simulink model "simple_line_follower_simulation_new"  (R2020a)
settings: Solver=FixedStepAuto  StartTime=0.0  StopTime=5  FixedStep=0.01  RelTol=1e-3
values from neighbouring files (symbols this model uses):
  axleLength = 0.0672    [robotParameters_maze.m]
  J = 0.0001    [robotParameters_maze.m]
  Kb = 0.190    (= 0.19)    [robotParameters_maze.m]
  Kf = 0.000025    (= 2.5e-05)    [robotParameters_maze.m]
  Km = 0.084    [robotParameters_maze.m]
  L = 0.5    [robotParameters_maze.m]
  mapForSim =     [maze_map.mat]    (also in oval_line_map.mat)
  motorIP = [-12 -11.9 -11.8 -11.7 -11.6 -11.5 -11.4 -11.3 -11.2 -11.1 -11 -10.9 ... (241 elements, 1x241)]    [motorLUT.mat]
  motorSP = [-62.7865560716 -62.2538153955 -61.7309054619 -61.2077148683 -60.684548166 -60.1613790322 -59.6382101464 -59.1150412352 -58.5918723266 -58.0687034178 -57.545534509 -57.0223656001 ... (241 elements, 1x241)]    [motorLUT.mat]
  R = 16    [robotParameters_maze.m]
  wheelR = 0.017    [robotParameters_maze.m]
undefined symbols (not defined in the file or in its folder): DiscIntNeverNeededParam, lineLength
libraries: mobileRoboticsTrainingLib x2, eeGeneralControl x1, simulink x1, sldrtlib x1
settings Model: Creator=RAJENDRA PHUTANE  LastModifiedBy=RAJENDRA PHUTANE

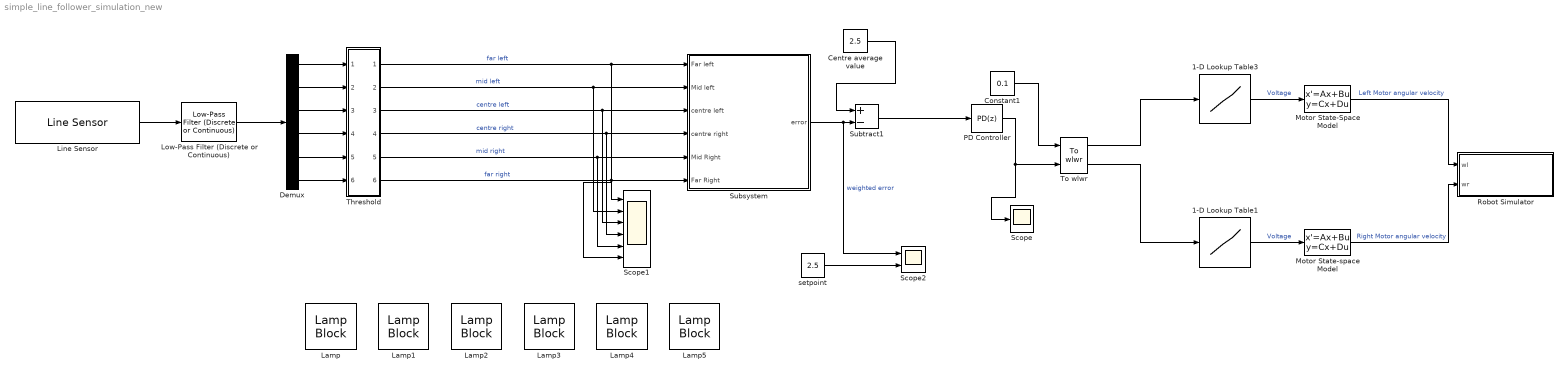
== system simple_line_follower_simulation_new ==
  1-D Lookup Table1 : Lookup_n-D  NumberOfTableDimensions=1  BreakpointsForDimension1=motorSP  Table=motorIP  ExtrapMethod=Clip  InternalRulePriority=Speed  RndMeth=Simplest  InputSameDT=on
  1-D Lookup Table3 : Lookup_n-D  NumberOfTableDimensions=1  BreakpointsForDimension1=motorSP  Table=motorIP  ExtrapMethod=Clip  InternalRulePriority=Speed  RndMeth=Simplest  InputSameDT=on
  Centre average value : Constant  Value=2.5
  Constant1 : Constant  Value=0.1
  Demux : Demux  Outputs=6
  Lamp{,1..5} (6 alike) : LampBlock
  Line Sensor : mobileRoboticsTrainingLib/Line Sensor  mapVariable=mapForSim  envVal=0  lineVal=1000  sensOff=[0.075 0.045;0.075 0.027;0.075 0.009;0.075 -0.009;0.075 -0.027;0.075 -0.045]
      settings: SourceProductName=Mobile Robotics Training Library
  Low-Pass Filter (Discrete or Continuous) : eeGeneralControl/Low-Pass Filter (Discrete or Continuous)  K=1  T=0.2  B=inf  A=-inf  init_option=Inherited from block input  x0=0  Ts=0.01
  Motor State-Space Model : StateSpace  A=[-Kf/J Km/J; -Kb/L -R/L]  B=[0; 1/L]  C=[1 0]  D=[0]  InitialCondition=0
  Motor State-space Model : StateSpace  A=[-Kf/J Km/J; -Kb/L -R/L]  B=[0; 1/L]  C=[1 0]  D=[0]  InitialCondition=0
  PD Controller : simulink/Continuous/PID Controller  Controller=PD  Form=Parallel  TimeDomain=Discrete-time  UseExternalTs=off  SampleTime=-1  IntegratorMethod=Forward Euler  FilterMethod=Forward Euler  ControllerParametersSource=internal  P=0.6  I=-100  D=1e-5  UseFilter=on  N=100  TunerSelectOption=Transfer Function Based (PID Tuner App)  InitialConditionSource=internal  InitialConditionForIntegrator=0  InitialConditionForFilter=0  DifferentiatorICPrevScaledInput=0  ExternalReset=none  TrackingMode=off  Kt=1  LimitOutput=off  UpperSaturationLimit=inf  LowerSaturationLimit=-inf  LinearizeAsGain=on  AntiWindupMode=none  Kb=1  POutMin=[]  POutMax=[]  IOutMin=[]  IOutMax=[]  DOutMin=[]  DOutMax=[]  NOutMin=[]  NOutMax=[]  SumOutMin=[]  SumOutMax=[]  SaturationOutMin=[]  SaturationOutMax=[]  PParamMin=[]  PParamMax=[]  IParamMin=[]  IParamMax=[]  DParamMin=[]  DParamMax=[]  NParamMin=[]  NParamMax=[]  KbParamMin=[]  KbParamMax=[]  KtParamMin=[]  KtParamMax=[]  KbOutMin=[]  KbOutMax=[]  KtOutMin=[]  KtOutMax=[]  IntegratorOutMin=[]  IntegratorOutMax=[]  FilterOutMin=[]  FilterOutMax=[]  SumI1OutMin=[]  SumI1OutMax=[]  SumI2OutMin=[]  SumI2OutMax=[]  SumI3OutMin=[]  SumI3OutMax=[]  SumI4OutMin=[]  SumI4OutMax=[]  SumDOutMin=[]  SumDOutMax=[]  DifferentiatorOutMin=[]  DifferentiatorOutMax=[]  FilterDiffOutCoefMin=[]  FilterDiffOutCoefMax=[]  ReciprocalOutMin=[]  ReciprocalOutMax=[]  SumDenOutMin=[]  SumDenOutMax=[]  SumNumOutMin=[]  SumNumOutMax=[]  DivideOutMin=[]  DivideOutMax=[]  UdiffTsProdOutMin=[]  UdiffTsProdOutMax=[]  NTsProdOutMin=[]  NTsProdOutMax=[]  UintegralTsProdOutMin=[]  UintegralTsProdOutMax=[]  UngainTsProdOutMin=[]  UngainTsProdOutMax=[]  IntegratorContinuousStateAttributes=''  IntegratorStateMustResolveToSignalObject=off  IntegratorRTWStateStorageClass=Auto  FilterContinuousStateAttributes=''  FilterStateMustResolveToSignalObject=off  FilterRTWStateStorageClass=Auto  ParallelPVariant=InternalParameters  IdealPVariant=Disabled  IVariant=Disabled  DVariant=InternalParameters  IntegratorVariant=Disabled  SatVariant=Disabled  AWVariant=Disabled  PCopyVariant=Disabled  TRVariant=Disabled  FdbkBlocksVariant=Forward  IdealPFdbkVariant=Disabled  SatFdbkVariant=Disabled  DerivativeFilterVariant=ForwardEulerFilter  NVariant=InternalParameters  NCopyVariant=Disabled  FilterICVariant=InternalICsFilter  IntegratorICVariant=Disabled  ExternalResetVariant=Disabled  TRSumVariant=Passthrough  SumFdbkVariant=Disabled  SumVariant=Sum_PD  TsampFilterVariant=InternalTs  TsampNgainVariant=Passthrough  TsampIntegralVariant=Disabled_SignalSpec  InitialConditionSetting=Output
  Robot Simulator : Subsystem  Priority=99  mask(Robot Simulator){mapVar=mapForSim, startX=1.6679, startY=0.46334, startTheta=90, axleLength=axleLength, wheelR=wheelR}
      mask prompts: mapVar "Map Variable"; startX "Start X (m)"; startY "Start Y (m)"; startTheta "Theta (deg)"; axleLength "Axle Length (m)"; wheelR "Wheel Radius (m)"
      mask help: Configure robot simulator to use custom simulation maps and simulate closed-loop mobile robotics systems along with appropriate sensor simulation blocks.
      mask init:
      | set_param(bdroot,'SolverType','Fixed-Step');
      | set_param(bdroot,'Solver','FixedStepAuto');
      | 
      | if (exist('Ts'))
      |     set_param(bdroot,'FixedStep','Ts');
      | else
      |     set_param(bdroot,'FixedStep','0.01');
      | end
      | h = findobj('Name','Robot Simulator');
      | if ~isempty(h)
      |     close (h);
      | end
      | setupRobotSim();
      mask Help: web('Robot Simulator.htm')
      mask DialogControl mapCont Prompt: Map Setup
      mask DialogControl initPosCont Prompt: Initial Position
      mask DialogControl setPos Prompt: Set position interactively
      mask DialogControl setPos Callback:
      | %% Set starting point
      | setStartingPoint();
      mask DialogControl initOrientation Prompt: Initial Orientation
      mask DialogControl robotCharCont Prompt: Robot Characteristics
      mask Display: disp('Robot Simulator')
  Scope : Scope
  Scope1 : Scope  NumInputPorts=6
  Scope2 : Scope  NumInputPorts=2
  Subsystem : Subsystem
  Subtract1 : Sum  Inputs=+-
  Threshold : Subsystem
  To wlwr : mobileRoboticsTrainingLib/To wlwr  axleLength=axleLength  wheelR=wheelR
  setpoint : Constant  Value=2.5
  wires:
  Line Sensor/1 -> Low-Pass Filter (Discrete or Continuous)/1
  Threshold/1(Out1) -> Scope1/1, Subsystem/1(Far left)  "far left"
  Threshold/2(Out2) -> Subsystem/2(Mid left), Scope1/2  "mid left"
  Threshold/3(Out3) -> Subsystem/3(centre left), Scope1/3  "centre left"
  Threshold/4(Out4) -> Subsystem/4(centre right), Scope1/4  "centre right"
  Threshold/5(Out5) -> Subsystem/5(Mid Right), Scope1/5  "mid right"
  Threshold/6(Out6) -> Scope1/6, Subsystem/6(Far Right)  "far right"
  Demux/1 -> Threshold/1(In1)
  Demux/2 -> Threshold/2(In2)
  Demux/6 -> Threshold/6(In6)
  Demux/5 -> Threshold/5(In5)
  Demux/4 -> Threshold/4(In4)
  Demux/3 -> Threshold/3(In3)
  Constant1/1 -> To wlwr/1
  PD Controller/1 -> Scope/1, To wlwr/2
  Centre average value/1 -> Subtract1/1
  Subsystem/1(error) -> Scope2/1, Subtract1/2  "weighted error"
  Subtract1/1 -> PD Controller/1
  To wlwr/2 -> 1-D Lookup Table1/1
  To wlwr/1 -> 1-D Lookup Table3/1
  Low-Pass Filter (Discrete or Continuous)/1 -> Demux/1
  Motor State-space Model/1 -> Robot Simulator/2(wr)  "Right Motor angular velocity"
  Motor State-Space Model/1 -> Robot Simulator/1(wl)  "Left Motor angular velocity"
  1-D Lookup Table3/1 -> Motor State-Space Model/1  "Voltage"
  1-D Lookup Table1/1 -> Motor State-space Model/1  "Voltage"
  setpoint/1 -> Scope2/2

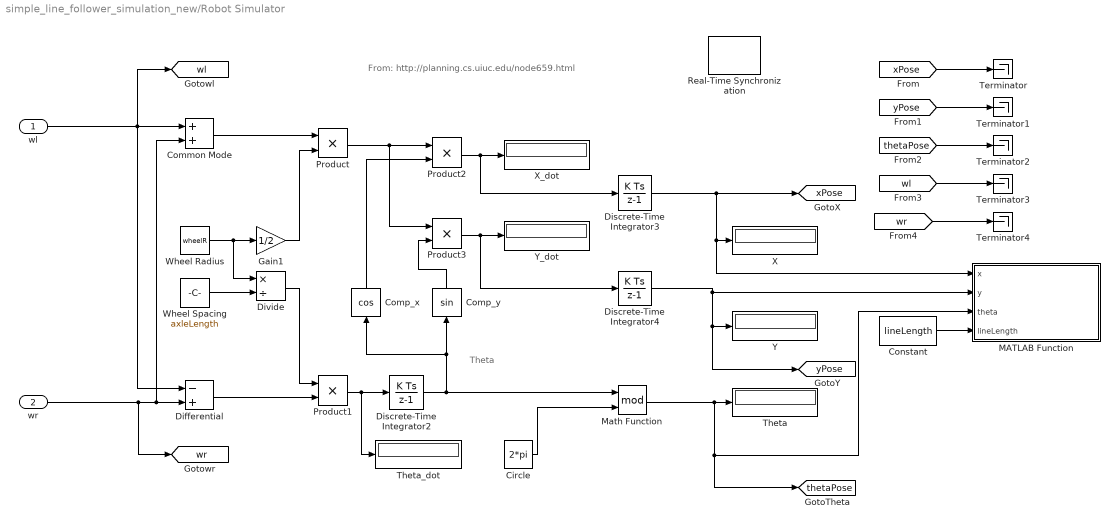
== system simple_line_follower_simulation_new/Robot Simulator ==
  note: Theta
  note: From: http://planning.cs.uiuc.edu/node659.html
  wl : Inport
  wr : Inport  Port=2
  Circle : Constant  Value=2*pi
  Common Mode : Sum
  Comp_x : Trigonometry  Operator=cos
  Comp_y : Trigonometry
  Constant : Constant  Value=lineLength
  Differential : Sum  Inputs=-+
  Discrete-Time Integrator2 : DiscreteIntegrator  InitialCondition=startTheta*(pi/180)  SampleTime=-1  ICPrevOutput=DiscIntNeverNeededParam  ICPrevScaledInput=DiscIntNeverNeededParam
  Discrete-Time Integrator3 : DiscreteIntegrator  InitialCondition=startX  SampleTime=-1  ICPrevOutput=DiscIntNeverNeededParam  ICPrevScaledInput=DiscIntNeverNeededParam
  Discrete-Time Integrator4 : DiscreteIntegrator  InitialCondition=startY  SampleTime=-1  ICPrevOutput=DiscIntNeverNeededParam  ICPrevScaledInput=DiscIntNeverNeededParam
  Divide : Product  Inputs=*/
  Gain1 : Gain  Gain=1/2
  MATLAB Function : MATLAB Function  TreatAsAtomicUnit=on
  Math Function : Math  Operator=mod  SignedPower=on  SaturateOnIntegerOverflow=on
  Product{,1..3} (4 alike) : Product  RndMeth=Zero
  Real-Time Synchronization : sldrtlib/Real-Time Synchronization  SampleTime=0.01  MaxMissedTicks=100  ShowMissedTicks=off  YieldWhenWaiting=off
  Terminator{,1..4} (5 alike) : Terminator
  Theta : Display
  Theta_dot : Display
  Wheel Radius : Constant  Value=wheelR
  Wheel Spacing : Constant  Value=axleLength
  X : Display
  X_dot : Display
  Y : Display
  Y_dot : Display
  tag scope: thetaPose=global, wl=global, wr=global, xPose=global, yPose=global
  wires:
  [wr] -> Terminator4/1
  [wl] -> Terminator3/1
  Math Function/1 -> [thetaPose], MATLAB Function/3(theta), Theta/1
  Differential/1 -> Product1/2
  Comp_y/1 -> Product3/2
  Discrete-Time Integrator3/1 -> [xPose], MATLAB Function/1(x), X/1
  Product3/1 -> Discrete-Time Integrator4/1, Y_dot/1
  Discrete-Time Integrator4/1 -> Y/1, [yPose], MATLAB Function/2(y)
  Divide/1 -> Product1/1
  wr/1 -> [wr], Common Mode/2, Differential/2
  Discrete-Time Integrator2/1 -> Math Function/1, Comp_x/1, Comp_y/1
  wl/1 -> [wl], Common Mode/1, Differential/1
  Comp_x/1 -> Product2/2
  Product1/1 -> Discrete-Time Integrator2/1, Theta_dot/1
  Wheel Radius/1 -> Divide/1, Gain1/1
  Wheel Spacing/1 -> Divide/2
  Product2/1 -> Discrete-Time Integrator3/1, X_dot/1
  Gain1/1 -> Product/2
  Common Mode/1 -> Product/1
  Product/1 -> Product3/1, Product2/1
  Circle/1 -> Math Function/2
  Constant/1 -> MATLAB Function/4(lineLength)
  [xPose] -> Terminator/1
  [yPose] -> Terminator1/1
  [thetaPose] -> Terminator2/1

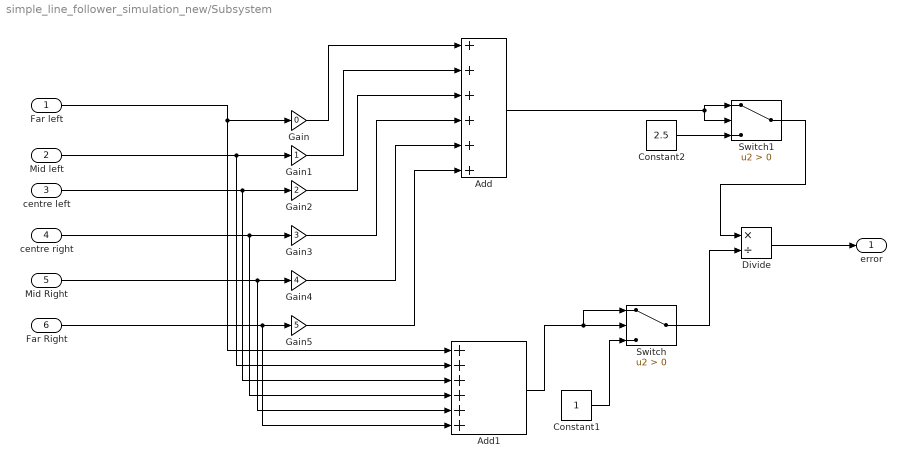
== system simple_line_follower_simulation_new/Subsystem ==
  Far left : Inport
  Mid left : Inport  Port=2
  centre left : Inport  Port=3
  centre right : Inport  Port=4
  Mid Right : Inport  Port=5
  Far Right : Inport  Port=6
  Add : Sum  Inputs=++++++
  Add1 : Sum  Inputs=++++++
  Constant1 : Constant
  Constant2 : Constant  Value=2.5
  Divide : Product  Inputs=*/
  Gain : Gain  Gain=0
  Gain1 : Gain
  Gain2 : Gain  Gain=2
  Gain3 : Gain  Gain=3
  Gain4 : Gain  Gain=4
  Gain5 : Gain  Gain=5
  Switch : Switch  Criteria=u2 > Threshold
  Switch1 : Switch  Criteria=u2 > Threshold
  error : Outport
  wires:
  Far left/1 -> Add1/1, Gain/1
  Gain5/1 -> Add/6
  centre left/1 -> Add1/3, Gain2/1
  Far Right/1 -> Add1/6, Gain5/1
  centre right/1 -> Add1/4, Gain3/1
  Divide/1 -> error/1
  Gain4/1 -> Add/5
  Gain1/1 -> Add/2
  Gain3/1 -> Add/4
  Add1/1 -> Switch/1, Switch/2
  Constant1/1 -> Switch/3
  Add/1 -> Switch1/1, Switch1/2
  Switch/1 -> Divide/2
  Gain/1 -> Add/1
  Mid Right/1 -> Add1/5, Gain4/1
  Gain2/1 -> Add/3
  Mid left/1 -> Add1/2, Gain1/1
  Constant2/1 -> Switch1/3
  Switch1/1 -> Divide/1

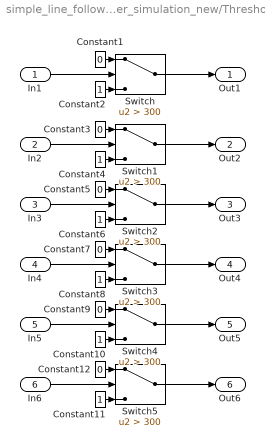
== system simple_line_follower_simulation_new/Threshold ==
  In1 : Inport
  In2 : Inport  Port=2
  In3 : Inport  Port=3
  In4 : Inport  Port=4
  In5 : Inport  Port=5
  In6 : Inport  Port=6
  Constant{1,3,5,7,9,12} (6 alike) : Constant  Value=0
  Constant{2,4,6,8,10..11} (6 alike) : Constant
  Switch{,1..5} (6 alike) : Switch  Criteria=u2 > Threshold  Threshold=300
  Out1 : Outport
  Out2 : Outport  Port=2
  Out3 : Outport  Port=3
  Out4 : Outport  Port=4
  Out5 : Outport  Port=5
  Out6 : Outport  Port=6
  wires:
  Constant2/1 -> Switch/3
  Constant1/1 -> Switch/1
  Switch/1 -> Out1/1
  In1/1 -> Switch/2
  In2/1 -> Switch1/2
  Switch1/1 -> Out2/1
  Constant3/1 -> Switch1/1
  Constant4/1 -> Switch1/3
  Constant6/1 -> Switch2/3
  Constant5/1 -> Switch2/1
  Switch2/1 -> Out3/1
  In3/1 -> Switch2/2
  In4/1 -> Switch3/2
  Switch3/1 -> Out4/1
  Constant7/1 -> Switch3/1
  Constant8/1 -> Switch3/3
  Constant10/1 -> Switch4/3
  Constant9/1 -> Switch4/1
  Switch4/1 -> Out5/1
  In5/1 -> Switch4/2
  In6/1 -> Switch5/2
  Switch5/1 -> Out6/1
  Constant12/1 -> Switch5/1
  Constant11/1 -> Switch5/3

== matlab function simple_line_follower_simulation_new/Robot Simulator/MATLAB Function ==
  data: x input; y input; theta input; lineLength input
function plotRobot(x,y,theta,lineLength)
% Get plot details
coder.extrinsic('evalin','plot')
ph1 = evalin('base','PlotHandle1');
ph2 = evalin('base','PlotHandle2');

% Find length orientation line
xp = [x x+lineLength*cos(theta)];
yp = [y y+lineLength*sin(theta)];

% Plot robot
set(ph1,'xdata',xp,'ydata',yp);
set(ph2,'xdata',x,'ydata',y);
drawnow('limitrate')
